simulink model "BatterySupply"  (R2018a)
settings: Solver=FixedStepDiscrete  StartTime=0.0  StopTime=50.0  FixedStep=0.5  RelTol=1e-3
libraries: arduinolib x8, simulink x2
settings Model: Creator=fabricek  LastModifiedBy=fabricek

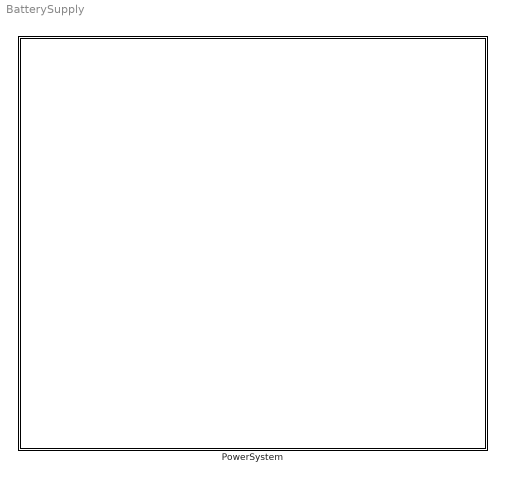
== system BatterySupply ==
  PowerSystem : Subsystem

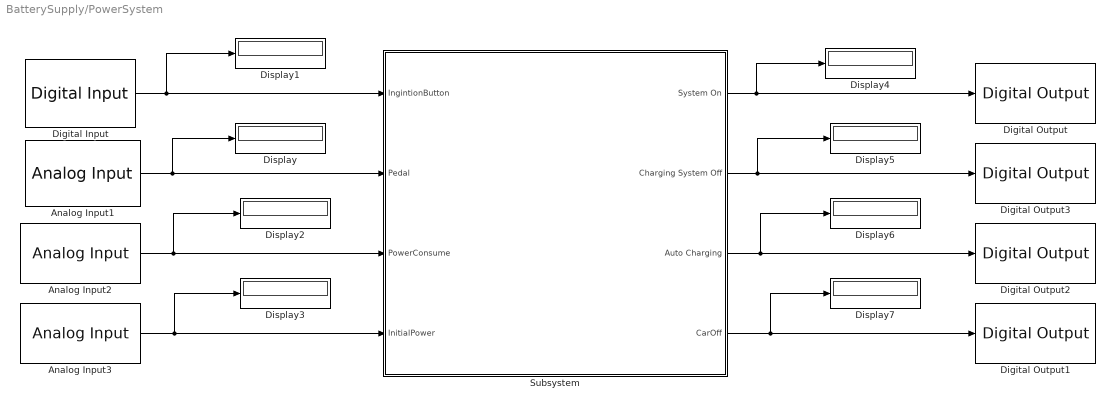
== system BatterySupply/PowerSystem ==
  Analog Input1 : arduinolib/Analog Input  pinNumber=2  ReadResultsOnly=off  ConversionTriggerSource=Software  ExternalTriggerType=uint32(0)  OutputDataType=uint16  EnableConversionCompleteNotify=off  EnableOuputStatus=off  SampleTime=1  blockPlatform=arduino
  Analog Input2 : arduinolib/Analog Input  pinNumber=1  ReadResultsOnly=off  ConversionTriggerSource=Software  ExternalTriggerType=uint32(0)  OutputDataType=uint16  EnableConversionCompleteNotify=off  EnableOuputStatus=off  SampleTime=1  blockPlatform=arduino
  Analog Input3 : arduinolib/Analog Input  pinNumber=0  ReadResultsOnly=off  ConversionTriggerSource=Software  ExternalTriggerType=uint32(0)  OutputDataType=uint16  EnableConversionCompleteNotify=off  EnableOuputStatus=off  SampleTime=1  blockPlatform=arduino
  Digital Input : arduinolib/Digital Input  pinNumber=13  sampleTime=0.1  blockPlatform=arduino
      link override Digital Input: SampleTime=1
      settings: SourceProductName=Simulink Support Package for Arduino Hardware
  Digital Output : arduinolib/Digital Output  pinNumber=9  blockPlatform=arduino
  Digital Output1 : arduinolib/Digital Output  pinNumber=2  blockPlatform=arduino
  Digital Output2 : arduinolib/Digital Output  pinNumber=4  blockPlatform=arduino
  Digital Output3 : arduinolib/Digital Output  pinNumber=7  blockPlatform=arduino
  Display{,1..7} (8 alike) : Display
  Subsystem : Subsystem
  wires:
  Analog Input1/1 -> Subsystem/2(Pedal), Display/1
  Subsystem/1(System On) -> Digital Output/1, Display4/1
  Analog Input2/1 -> Subsystem/3(PowerConsume), Display2/1
  Subsystem/3(Auto Charging) -> Digital Output2/1, Display6/1
  Analog Input3/1 -> Subsystem/4(InitialPower), Display3/1
  Digital Input/1 -> Subsystem/1(IngintionButton), Display1/1
  Subsystem/2(Charging System Off) -> Digital Output3/1, Display5/1
  Subsystem/4(CarOff) -> Digital Output1/1, Display7/1

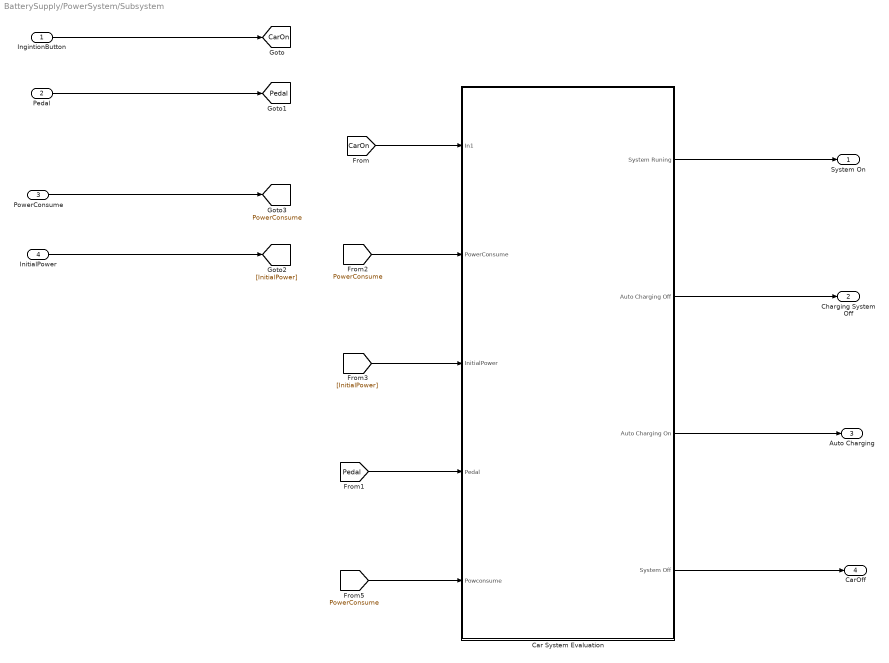
== system BatterySupply/PowerSystem/Subsystem ==
  IngintionButton : Inport
  Pedal : Inport  Port=2
  PowerConsume : Inport  Port=3
  InitialPower : Inport  Port=4
  Car System Evaluation : Subsystem
  System On : Outport
  Charging System Off : Outport  Port=2
  Auto Charging : Outport  Port=3
  CarOff : Outport  Port=4
  tag scope: CarOn=global, Pedal=global, PowerConsume=global
  wires:
  IngintionButton/1 -> [CarOn]
  Pedal/1 -> [Pedal]
  PowerConsume/1 -> [PowerConsume]
  InitialPower/1 -> [InitialPower]
  [CarOn] -> Car System Evaluation/1(In1)
  Car System Evaluation/4(System Off) -> CarOff/1
  Car System Evaluation/1(System Runing) -> System On/1
  Car System Evaluation/2(Auto Charging Off) -> Charging System Off/1
  Car System Evaluation/3(Auto Charging On) -> Auto Charging/1
  [Pedal] -> Car System Evaluation/4(Pedal)
  [PowerConsume] -> Car System Evaluation/2(PowerConsume)
  [PowerConsume] -> Car System Evaluation/5(Powconsume)
  [InitialPower] -> Car System Evaluation/3(InitialPower)

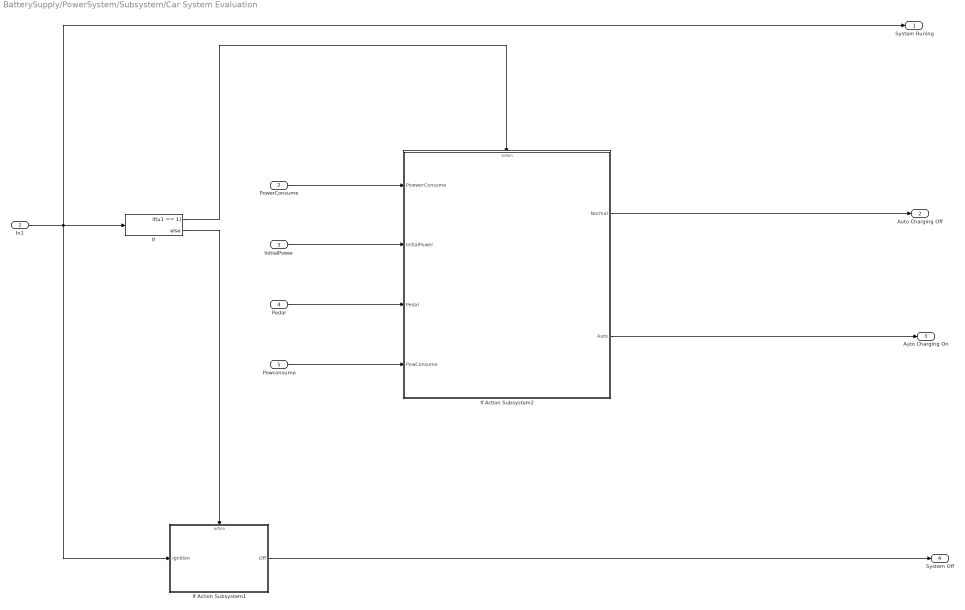
== system BatterySupply/PowerSystem/Subsystem/Car System Evaluation ==
  In1 : Inport
  PowerConsume : Inport  Port=2
  InitialPower : Inport  Port=3
  Pedal : Inport  Port=4  LockScale=on
  Powconsume : Inport  Port=5
  If : If  IfExpression=u1 == 1
  If Action Subsystem1 : Subsystem  TreatAsAtomicUnit=on
  If Action Subsystem2 : Subsystem  TreatAsAtomicUnit=on
  System Runing : Outport
  Auto Charging Off : Outport  Port=2
  Auto Charging On : Outport  Port=3
  System Off : Outport  Port=4
  wires:
  If Action Subsystem1/1(Off) -> System Off/1
  In1/1 -> If/1, System Runing/1, If Action Subsystem1/1(Ignition)
  If Action Subsystem2/1(Normal) -> Auto Charging Off/1
  If Action Subsystem2/2(Auto) -> Auto Charging On/1
  If/1 -> If Action Subsystem2/Action
  If/2 -> If Action Subsystem1/Action
  PowerConsume/1 -> If Action Subsystem2/1(PowwerConsume)
  InitialPower/1 -> If Action Subsystem2/2(InitialPower)
  Pedal/1 -> If Action Subsystem2/3(Pedal)
  Powconsume/1 -> If Action Subsystem2/4(PowConsume)

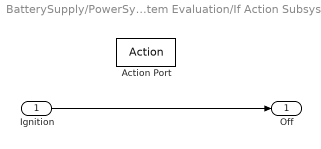
== system BatterySupply/PowerSystem/Subsystem/Car System Evaluation/If Action Subsystem1 ==
  Ignition : Inport
  Action Port : ActionPort  ActionType=else
  Off : Outport
  wires:
  Ignition/1 -> Off/1

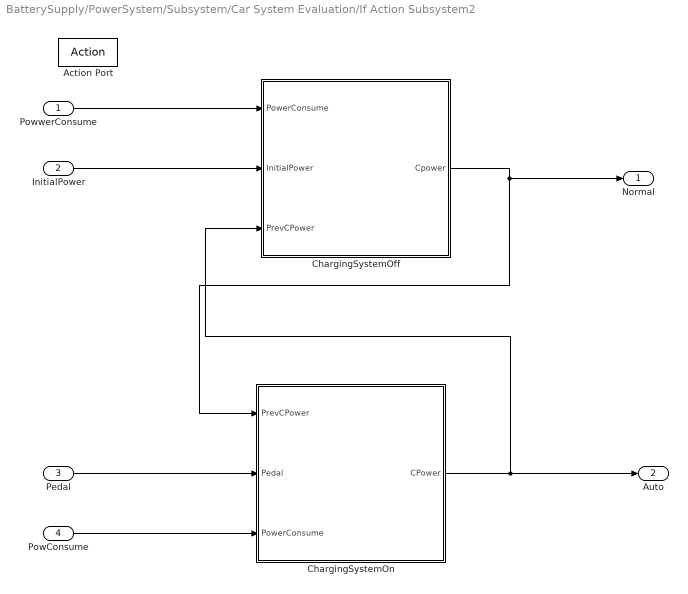
== system BatterySupply/PowerSystem/Subsystem/Car System Evaluation/If Action Subsystem2 ==
  PowwerConsume : Inport
  InitialPower : Inport  Port=2
  Pedal : Inport  Port=3
  PowConsume : Inport  Port=4
  Action Port : ActionPort  ActionType=then
  ChargingSystemOff : Subsystem  TreatAsAtomicUnit=on
  ChargingSystemOn : Subsystem  TreatAsAtomicUnit=on
  Normal : Outport
  Auto : Outport  Port=2
  wires:
  PowConsume/1 -> ChargingSystemOn/3(PowerConsume)
  ChargingSystemOn/1(CPower) -> ChargingSystemOff/3("   PrevCPower"), Auto/1
  InitialPower/1 -> ChargingSystemOff/2(InitialPower)
  Pedal/1 -> ChargingSystemOn/2(Pedal)
  ChargingSystemOff/1(Cpower) -> ChargingSystemOn/1("   PrevCPower"), Normal/1
  PowwerConsume/1 -> ChargingSystemOff/1(PowerConsume)

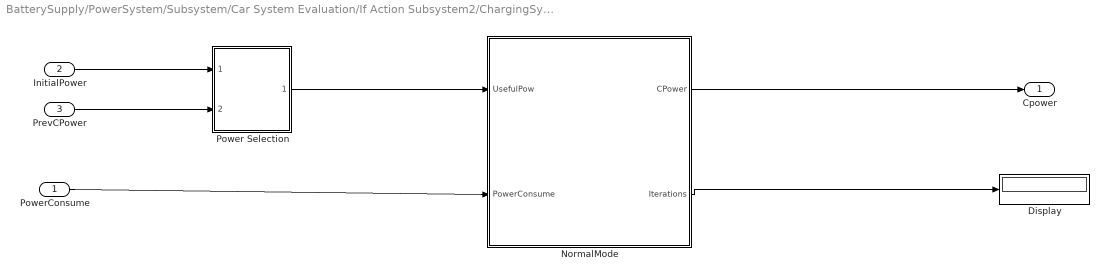
== system BatterySupply/PowerSystem/Subsystem/Car System Evaluation/If Action Subsystem2/ChargingSystemOff ==
  PowerConsume : Inport
  InitialPower : Inport  Port=2
  "   PrevCPower" : Inport  Port=3
  Display : Display
  NormalMode : Subsystem
  Power Selection : Subsystem
  Cpower : Outport
  wires:
  InitialPower/1 -> Power Selection/1(InitialPower)
  "   PrevCPower"/1 -> Power Selection/2(RPower)
  Power Selection/1(UsefulPower) -> NormalMode/1(UsefulPow)
  PowerConsume/1 -> NormalMode/2(PowerConsume)
  NormalMode/1(CPower) -> Cpower/1
  NormalMode/2(Iterations) -> Display/1

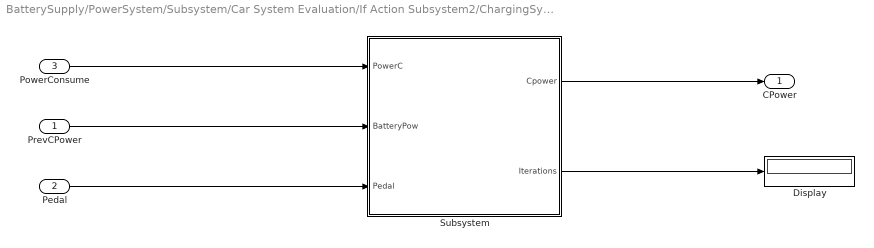
== system BatterySupply/PowerSystem/Subsystem/Car System Evaluation/If Action Subsystem2/ChargingSystemOn ==
  "   PrevCPower" : Inport
  Pedal : Inport  Port=2
  PowerConsume : Inport  Port=3
  Display : Display
  Subsystem : Subsystem
  CPower : Outport
  wires:
  PowerConsume/1 -> Subsystem/1("   PowerC")
  "   PrevCPower"/1 -> Subsystem/2(BatteryPow)
  Pedal/1 -> Subsystem/3(Pedal)
  Subsystem/1(Cpower) -> CPower/1
  Subsystem/2(Iterations) -> Display/1

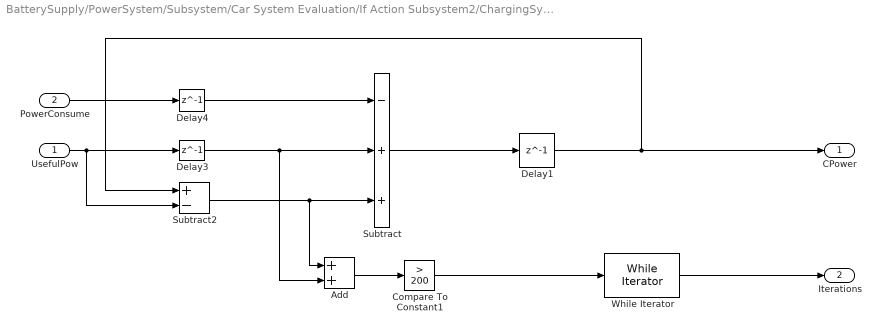
== system BatterySupply/PowerSystem/Subsystem/Car System Evaluation/If Action Subsystem2/ChargingSystemOff/NormalMode ==
  UsefulPow : Inport
  PowerConsume : Inport  Port=2
  Add : Sum
  Compare To Constant1 : simulink/Logic and Bit Operations/Compare To Constant  relop=>  const=200  OutDataTypeStr=boolean
  Delay1 : Delay  DelayLength=1
  Delay3 : Delay  DelayLength=1
  Delay4 : Delay  DelayLength=1
  Subtract : Sum  Inputs=-++
  Subtract2 : Sum  Inputs=+-
  While Iterator : WhileIterator  MaxIters=20  WhileBlockType=do-while  ShowIterationPort=on
  CPower : Outport
  Iterations : Outport  Port=2
  wires:
  UsefulPow/1 -> Delay3/1, Subtract2/2
  Add/1 -> Compare To Constant1/1
  Compare To Constant1/1 -> While Iterator/1
  While Iterator/1 -> Iterations/1
  Subtract2/1 -> Add/1, Subtract/3
  Delay3/1 -> Add/2, Subtract/2
  Subtract/1 -> Delay1/1
  Delay1/1 -> Subtract2/1, CPower/1
  PowerConsume/1 -> Delay4/1
  Delay4/1 -> Subtract/1

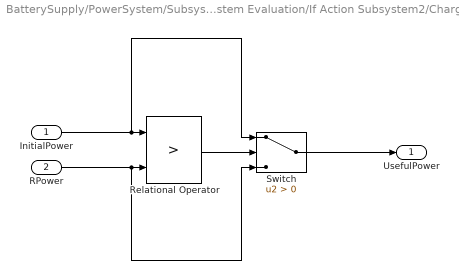
== system BatterySupply/PowerSystem/Subsystem/Car System Evaluation/If Action Subsystem2/ChargingSystemOff/Power Selection ==
  InitialPower : Inport
  RPower : Inport  Port=2
  Relational Operator : RelationalOperator  Operator=>  OutDataTypeStr=boolean  RndMeth=Simplest
  Switch : Switch  Criteria=u2 > Threshold
  UsefulPower : Outport
  wires:
  Relational Operator/1 -> Switch/2
  RPower/1 -> Switch/3, Relational Operator/2
  InitialPower/1 -> Switch/1, Relational Operator/1
  Switch/1 -> UsefulPower/1

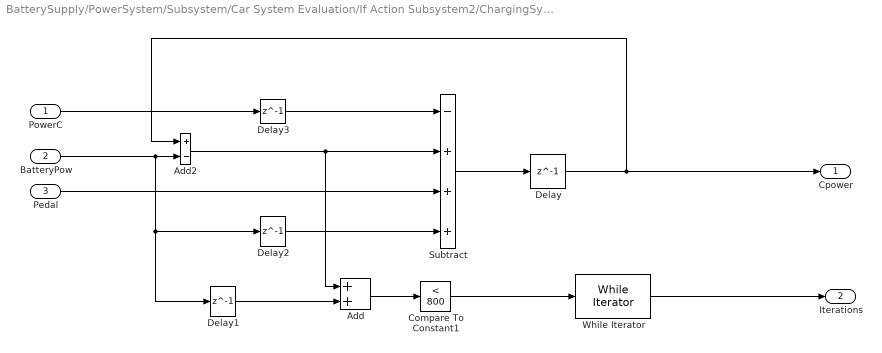
== system BatterySupply/PowerSystem/Subsystem/Car System Evaluation/If Action Subsystem2/ChargingSystemOn/Subsystem ==
  "   PowerC" : Inport
  BatteryPow : Inport  Port=2
  Pedal : Inport  Port=3
  Add : Sum
  Add2 : Sum  Inputs=+-
  Compare To Constant1 : simulink/Logic and Bit Operations/Compare To Constant  relop=<  const=800  OutDataTypeStr=boolean
  Delay{,1..3} (4 alike) : Delay  DelayLength=1
  Subtract : Sum  Inputs=-+++
  While Iterator : WhileIterator  MaxIters=20  WhileBlockType=do-while  ShowIterationPort=on
  Cpower : Outport
  Iterations : Outport  Port=2
  wires:
  BatteryPow/1 -> Add2/2, Delay1/1, Delay2/1
  Add2/1 -> Add/1, Subtract/2
  Compare To Constant1/1 -> While Iterator/1
  While Iterator/1 -> Iterations/1
  Add/1 -> Compare To Constant1/1
  Subtract/1 -> Delay/1
  Pedal/1 -> Subtract/3
  Delay/1 -> Add2/1, Cpower/1
  Delay1/1 -> Add/2
  Delay2/1 -> Subtract/4
  "   PowerC"/1 -> Delay3/1
  Delay3/1 -> Subtract/1
